simulink model "model_for_IM_with_ITSC_fault"  (R2016a)
settings: Solver=VariableStepAuto  StartTime=0.0  StopTime=2  FixedStep=2e-6  MaxStep=2e-6  RelTol=1e-6
libraries: powerlib x34, powerlib_meascontrol x1
settings Model: Creator=Pietro  LastModifiedBy=silker
settings SolverCC: ZeroCrossControl=DisableAll
settings DataIOCC: LimitDataPoints=on  SaveFormat=Array  SignalLoggingSaveFormat=ModelDataLogs
settings OptimizationCC: ExpressionDepthLimit=2147483647  InitFltsAndDblsToZero=on
settings DebuggingCC: SaveWithParameterizedLinksMsg=none  UnderspecifiedInitializationDetection=Classic  MergeDetectMultiDrivingBlocksExec=none  SignalResolutionControl=TryResolveAllWithWarning  SolverPrmCheckMsg=warning  MultiTaskDSMMsg=warning  MultiTaskCondExecSysMsg=none  FcnCallInpInsideContextMsg=UseLocalSettings  StateNameClashWarn=warning
settings HardwareCC: ProdBitPerPointer=32  ProdLargestAtomicFloat=None  ProdIntDivRoundTo=Undefined  ProdEndianess=Unspecified  ProdWordSize=32  ProdHWDeviceType=32-bit Generic
settings ModelReferenceCC: PropagateSignalLabelsOutOfModel=off
settings GRTTargetCC: TargetFcnLib=ansi_tfl_tmw.mat  CombineOutputUpdateFcns=off  GRTInterface=on
settings ConfigComp: CovModelRefEnable=Off

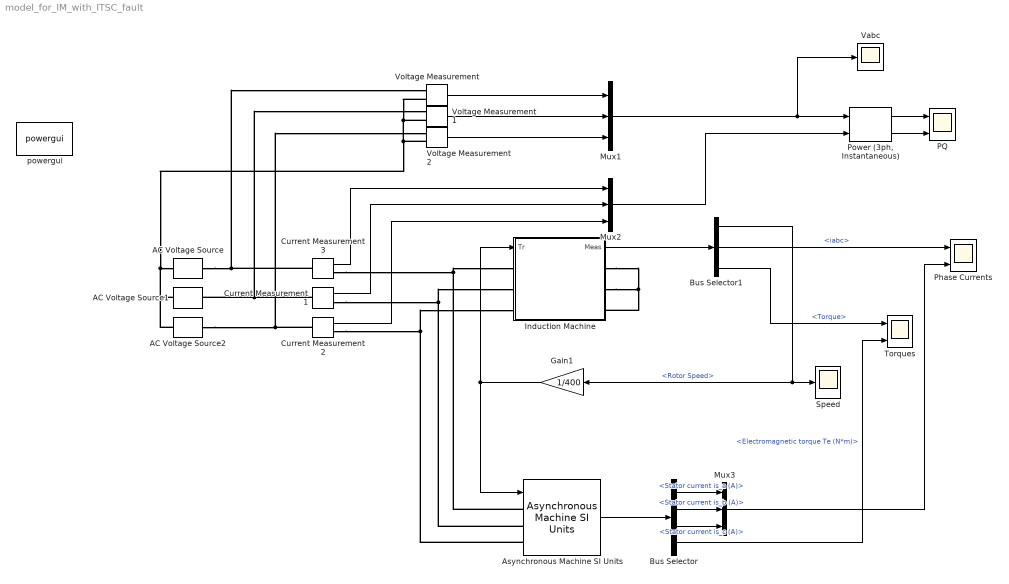
== system model_for_IM_with_ITSC_fault ==
  AC Voltage Source : powerlib/Electrical Sources/AC Voltage Source  Amplitude=80  Phase=0  Frequency=50  SampleTime=-1  Measurements=None  BusType=swing  Pref=10e3  Qref=0  Qmin=-inf  Qmax=+inf
  AC Voltage Source1 : powerlib/Electrical Sources/AC Voltage Source  Amplitude=80  Phase=240  Frequency=50  SampleTime=-1  Measurements=None  BusType=swing  Pref=10e3  Qref=0  Qmin=-inf  Qmax=+inf
  AC Voltage Source2 : powerlib/Electrical Sources/AC Voltage Source  Amplitude=80  Phase=120  Frequency=50  SampleTime=-1  Measurements=None  BusType=swing  Pref=10e3  Qref=0  Qmin=-inf  Qmax=+inf
  Asynchronous Machine SI Units : powerlib/Machines/Asynchronous Machine SI Units  RotorType=Squirrel-cage  PresetModel=No  MechanicalLoad=Torque Tm  ShowDetailedParameters=on  ReferenceFrame=Rotor  Units=SI  MeasurementBus=off  NominalParameters=[500 150 50]  Stator=[2.3 0.005]  Rotor=[3.1 0.001]  Cage1=[0.4155 0.002066]  Cage2=[0.4168 0.0003495]  Lm=0.090  Mechanical=[0.005 0.0000001 1]  PolePairs=2  InitialConditions=[1 0 0 0 0 0 0 0]  SimulateSaturation=off  Saturation=[14.03593122, 27.81365428, 53.79336849, 72.68890987, 97.98006896, 148.6815601, 215.7428561, 302.9841135, 428.7778367 ; 230, 322, 414, 460, 506, 552, 598, 644, 690]  LoadFlowParameters=1492000  TsPowergui=0  TsBlock=-1  IterativeModel=Trapezoidal non iterative  IterativeDiscreteModel=Trapezoidal non iterative  Pmec=1.492e+006
  Bus Selector : BusSelector  OutputSignals=Stator measurements.Stator current is_a (A),Stator measurements.Stator current is_b (A),Stator measurements.Stator current is_c (A),Mechanical.Electromagnetic torque Te (N*m)
  Bus Selector1 : BusSelector  OutputSignals=Rotor Speed,iabc,Torque
  Current Measurement1 : powerlib/Measurements/Current Measurement  PhasorSimulation=off  OutputType=Complex  PSBequivalent=0
  Current Measurement2 : powerlib/Measurements/Current Measurement  PhasorSimulation=off  OutputType=Complex  PSBequivalent=0
  Current Measurement3 : powerlib/Measurements/Current Measurement  PhasorSimulation=off  OutputType=Complex  PSBequivalent=0
  Gain1 : Gain  Gain=1/400
  Induction Machine : Subsystem  mask{Rs=2.3, Rr=3.1, Lm=0.090, Lls=0.005, Llr=0.001, PP=1, J=0.005, Kf=0.05, Rf=0.20}
      mask prompts: Kf "Fault Ratio"; Rf "Fault Resistance"
      mask help:
      | The initial VBR-based IM model by Pietro Tricoli,
      | Original file downloaded from:
      | https://www.mathworks.com/matlabcentral/fileexchange/53174-induction-machine-model
      mask init:
      | Lr=Llr+Lm;
      | Ls=Lls+Lm;
  Mux1 : Mux  Inputs=3
  Mux2 : Mux  Inputs=3
  Mux3 : Mux  Inputs=3
  PQ : Scope  NumInputPorts=2
  Phase Currents : Scope  NumInputPorts=2
  "Power (3ph, Instantaneous)" : powerlib_meascontrol/Measurements/Power (3ph, Instantaneous)
  Speed : Scope
  Torques : Scope  NumInputPorts=2
  Vabc : Scope
  Voltage Measurement : powerlib/Measurements/Voltage Measurement  PhasorSimulation=off  OutputType=Complex  PSBequivalent=0
  Voltage Measurement1 : powerlib/Measurements/Voltage Measurement  PhasorSimulation=off  OutputType=Complex  PSBequivalent=0
  Voltage Measurement2 : powerlib/Measurements/Voltage Measurement  PhasorSimulation=off  OutputType=Complex  PSBequivalent=0
  powergui : powerlib/powergui  Priority=1  SimulationMode=Discrete  SolverType=Tustin  SampleTime=2e-6  frequency=60  SPID=off  DisableSnubberDevices=off  DisableRonSwitches=off  DisableVfSwitches=off  SwTol=0  DisplayEquations=off  Interpol=off  ExternalGateDelay=off  methode=off  Ts=10  FunctionMessages=off  echomessages=off  HookPort=off  EnableUseOfTLC=off  x0status=blocks  frequencyindice=0  Pbase=100e6  ErrMax=1e-4  Iterations=50  UnitsV=kV  UnitsW=MW  buscounter=0  RestoreLinks=warning  ResistiveCurrentMeasurement=off  Frange=[0:2:500]  Ylog=off  Xlog=on  ShowGrid=off  save=off  variable=ZData  structure=0  ZoomFFT=off  StartTime=0.0  cycles=1  DisplayStyle=1  fundamental=60  FreqAxis=off  MaxFrequency=1000  frequencyindicesteady=1  RmsSteady=1  display=off
  wires:
  Voltage Measurement/1 -> Mux1/1
  Asynchronous Machine SI Units/1 -> Bus Selector/1
  Induction Machine/1(Meas) -> Bus Selector1/1
  Bus Selector1/1 -> Gain1/1, Speed/1  "<Rotor Speed>"
  Bus Selector1/2 -> Phase Currents/1  "<iabc>"
  Gain1/1 -> Asynchronous Machine SI Units/1, Induction Machine/1(Tr)
  Voltage Measurement1/1 -> Mux1/2
  Voltage Measurement2/1 -> Mux1/3
  Current Measurement3/1 -> Mux2/1
  Current Measurement1/1 -> Mux2/2
  Current Measurement2/1 -> Mux2/3
  Mux1/1 -> Vabc/1, "Power (3ph, Instantaneous)"/1
  Mux2/1 -> "Power (3ph, Instantaneous)"/2
  "Power (3ph, Instantaneous)"/1 -> PQ/1
  "Power (3ph, Instantaneous)"/2 -> PQ/2
  Bus Selector1/3 -> Torques/1  "<Torque>"
  Bus Selector/4 -> Torques/2  "<Electromagnetic torque Te (N*m)>"
  Bus Selector/2 -> Mux3/2  "<Stator current is_b (A)>"
  Bus Selector/1 -> Mux3/1  "<Stator current is_a (A)>"
  Bus Selector/3 -> Mux3/3  "<Stator current is_c (A)>"
  Mux3/1 -> Phase Currents/2
  connections:
  Asynchronous Machine SI Units/LConn2 -- Current Measurement1/RConn1 -- Induction Machine/LConn2
  Asynchronous Machine SI Units/LConn3 -- Current Measurement2/RConn1 -- Induction Machine/LConn3
  Asynchronous Machine SI Units/LConn1 -- Current Measurement3/RConn1 -- Induction Machine/LConn1
  Induction Machine/RConn1 -- Induction Machine/RConn3 -- Induction Machine/RConn2
  AC Voltage Source2/RConn1 -- Current Measurement2/LConn1 -- Voltage Measurement2/LConn1
  Current Measurement1/LConn1 -- AC Voltage Source1/RConn1 -- Voltage Measurement1/LConn1
  AC Voltage Source/RConn1 -- Current Measurement3/LConn1 -- Voltage Measurement/LConn1
  AC Voltage Source2/LConn1 -- AC Voltage Source1/LConn1 -- Voltage Measurement/LConn2 -- Voltage Measurement1/LConn2 -- Voltage Measurement2/LConn2 -- AC Voltage Source/LConn1

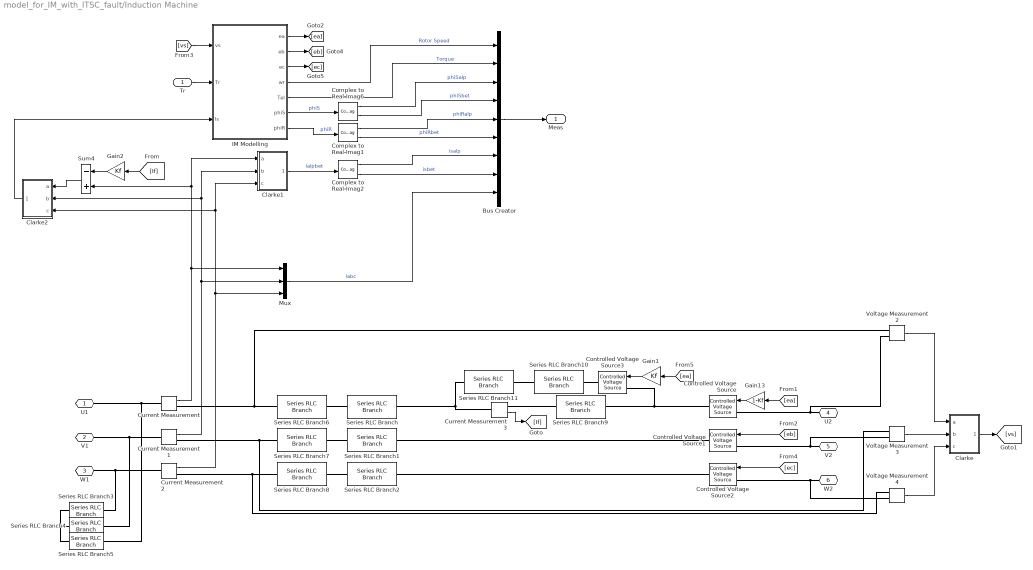
== system model_for_IM_with_ITSC_fault/Induction Machine ==
  Tr : Inport
  Bus Creator : BusCreator  Inputs=9
  Clarke : Subsystem
  Clarke1 : Subsystem
  Clarke2 : Subsystem
  Complex to Real-Imag1 : ComplexToRealImag
  Complex to Real-Imag2 : ComplexToRealImag
  Complex to Real-Imag6 : ComplexToRealImag
  Controlled Voltage Source{,1..3} (4 alike) : powerlib/Electrical Sources/Controlled Voltage Source  Initialize=on  Source_Type=AC  Amplitude=0  Phase=0  Frequency=0  Measurements=None
  Current Measurement{,1..3} (4 alike) : powerlib/Measurements/Current Measurement  PhasorSimulation=off  OutputType=Complex  PSBequivalent=0
  Gain1 : Gain  Gain=Kf
  Gain13 : Gain  Gain=1-Kf
  Gain2 : Gain  Gain=Kf
  IM Modelling : Subsystem
  Mux : Mux  Inputs=3
  Series RLC Branch : powerlib/Elements/Series RLC Branch  LConnTagsString=__new0  RConnTagsString=__new0  BranchType=L  Resistance=Rs  Inductance=Lls*(1-Kf)  SetiL0=off  InitialCurrent=0  Capacitance=1e-6  Setx0=off  InitialVoltage=0  Measurements=None
  Series RLC Branch1 : powerlib/Elements/Series RLC Branch  LConnTagsString=__new0  RConnTagsString=__new0  BranchType=L  Resistance=Rs  Inductance=Lls  SetiL0=on  InitialCurrent=0  Capacitance=1e-6  Setx0=off  InitialVoltage=0  Measurements=None
  Series RLC Branch10 : powerlib/Elements/Series RLC Branch  LConnTagsString=__new0  RConnTagsString=__new0  BranchType=L  Resistance=Rs  Inductance=Lls*Kf  SetiL0=off  InitialCurrent=0  Capacitance=1e-6  Setx0=off  InitialVoltage=0  Measurements=None
  Series RLC Branch11 : powerlib/Elements/Series RLC Branch  LConnTagsString=__new0  RConnTagsString=__new0  BranchType=R  Resistance=Rs*Kf  Inductance=Lls  SetiL0=off  InitialCurrent=0  Capacitance=1e-6  Setx0=off  InitialVoltage=0  Measurements=None
  Series RLC Branch2 : powerlib/Elements/Series RLC Branch  LConnTagsString=__new0  RConnTagsString=__new0  BranchType=L  Resistance=Rs  Inductance=Lls  SetiL0=on  InitialCurrent=0  Capacitance=1e-6  Setx0=off  InitialVoltage=0  Measurements=None
  Series RLC Branch3 : powerlib/Elements/Series RLC Branch  LConnTagsString=__new0  RConnTagsString=__new0  BranchType=R  Resistance=1e12  Inductance=Lls  SetiL0=off  InitialCurrent=0  Capacitance=1e-6  Setx0=off  InitialVoltage=0  Measurements=None
  Series RLC Branch4 : powerlib/Elements/Series RLC Branch  LConnTagsString=__new0  RConnTagsString=__new0  BranchType=R  Resistance=1e12  Inductance=Lls  SetiL0=off  InitialCurrent=0  Capacitance=1e-6  Setx0=off  InitialVoltage=0  Measurements=None
  Series RLC Branch5 : powerlib/Elements/Series RLC Branch  LConnTagsString=__new0  RConnTagsString=__new0  BranchType=R  Resistance=1e12  Inductance=Lls  SetiL0=off  InitialCurrent=0  Capacitance=1e-6  Setx0=off  InitialVoltage=0  Measurements=None
  Series RLC Branch6 : powerlib/Elements/Series RLC Branch  LConnTagsString=__new0  RConnTagsString=__new0  BranchType=R  Resistance=Rs*(1-Kf)  Inductance=Lls  SetiL0=off  InitialCurrent=0  Capacitance=1e-6  Setx0=off  InitialVoltage=0  Measurements=None
  Series RLC Branch7 : powerlib/Elements/Series RLC Branch  LConnTagsString=__new0  RConnTagsString=__new0  BranchType=R  Resistance=Rs  Inductance=Lls  SetiL0=on  InitialCurrent=0  Capacitance=1e-6  Setx0=off  InitialVoltage=0  Measurements=None
  Series RLC Branch8 : powerlib/Elements/Series RLC Branch  LConnTagsString=__new0  RConnTagsString=__new0  BranchType=R  Resistance=Rs  Inductance=Lls  SetiL0=on  InitialCurrent=0  Capacitance=1e-6  Setx0=off  InitialVoltage=0  Measurements=None
  Series RLC Branch9 : powerlib/Elements/Series RLC Branch  LConnTagsString=__new0  RConnTagsString=__new0  BranchType=R  Resistance=Rf  Inductance=Lls  SetiL0=on  InitialCurrent=0  Capacitance=1e-6  Setx0=off  InitialVoltage=0  Measurements=None
  Sum4 : Sum  Inputs=-+
  Voltage Measurement2 : powerlib/Measurements/Voltage Measurement  PhasorSimulation=off  OutputType=Complex  PSBequivalent=0
  Voltage Measurement3 : powerlib/Measurements/Voltage Measurement  PhasorSimulation=off  OutputType=Complex  PSBequivalent=0
  Voltage Measurement4 : powerlib/Measurements/Voltage Measurement  PhasorSimulation=off  OutputType=Complex  PSBequivalent=0
  U1 : PMIOPort  Port=1  Side=Left
  V1 : PMIOPort  Port=2  Side=Left
  W1 : PMIOPort  Port=3  Side=Left
  U2 : PMIOPort  Port=4  Side=Right
  V2 : PMIOPort  Port=5  Side=Right
  W2 : PMIOPort  Port=6  Side=Right
  Meas : Outport
  wires:
  Tr/1 -> IM Modelling/2(Tr)
  [eb] -> Controlled Voltage Source1/1
  Current Measurement1/1 -> Clarke2/2(b), Clarke1/2(b), Mux/2
  Current Measurement/1 -> Clarke1/1(a), Sum4/2, Mux/1
  IM Modelling/1(ea) -> [ea]
  IM Modelling/2(eb) -> [eb]
  IM Modelling/3(ec) -> [ec]
  IM Modelling/4(wr) -> Bus Creator/1  "Rotor Speed"
  [vs] -> IM Modelling/1(vs)
  Voltage Measurement2/1 -> Clarke/1(a)
  Voltage Measurement3/1 -> Clarke/2(b)
  Voltage Measurement4/1 -> Clarke/3(c)
  Clarke/1(alp bet) -> [vs]
  IM Modelling/5(Tel) -> Bus Creator/2  "Torque"
  Bus Creator/1 -> Meas/1
  Complex to Real-Imag6/1 -> Bus Creator/3  "phiSalp"
  Complex to Real-Imag6/2 -> Bus Creator/4  "phiSbet"
  IM Modelling/6(phiS) -> Complex to Real-Imag6/1  "phiS"
  IM Modelling/7(phiR) -> Complex to Real-Imag1/1  "phiR"
  Complex to Real-Imag1/1 -> Bus Creator/5  "phiRalp"
  Complex to Real-Imag1/2 -> Bus Creator/6  "phiRbet"
  Clarke1/1(alp bet) -> Complex to Real-Imag2/1  "ialpbet"
  Complex to Real-Imag2/1 -> Bus Creator/7  "isalp"
  Complex to Real-Imag2/2 -> Bus Creator/8  "isbet"
  Mux/1 -> Bus Creator/9  "iabc"
  Gain1/1 -> Controlled Voltage Source3/1
  Gain13/1 -> Controlled Voltage Source/1
  [ea] -> Gain13/1
  [ec] -> Controlled Voltage Source2/1
  Current Measurement3/1 -> [If]
  [ea] -> Gain1/1
  Current Measurement2/1 -> Clarke1/3(c), Clarke2/3(c), Mux/3
  Sum4/1 -> Clarke2/1(a)
  Gain2/1 -> Sum4/1
  [If] -> Gain2/1
  Clarke2/1(alp bet) -> IM Modelling/3(Is)
  connections:
  Controlled Voltage Source1/RConn1 -- Series RLC Branch1/RConn1
  U1/RConn1 -- Series RLC Branch5/RConn1 -- Current Measurement/LConn1
  Current Measurement1/LConn1 -- Series RLC Branch4/RConn1 -- V1/RConn1
  Current Measurement2/LConn1 -- Series RLC Branch3/RConn1 -- W1/RConn1
  V2/RConn1 -- Voltage Measurement3/LConn2 -- Controlled Voltage Source1/LConn1
  W2/RConn1 -- Voltage Measurement4/LConn2 -- Controlled Voltage Source2/LConn1
  Controlled Voltage Source/LConn1 -- Voltage Measurement2/LConn2 -- U2/RConn1
  Series RLC Branch3/LConn1 -- Series RLC Branch4/LConn1 -- Series RLC Branch5/LConn1
  Series RLC Branch8/RConn1 -- Series RLC Branch2/LConn1
  Series RLC Branch7/RConn1 -- Series RLC Branch1/LConn1
  Series RLC Branch6/RConn1 -- Series RLC Branch/LConn1
  Series RLC Branch6/LConn1 -- Current Measurement/RConn1 -- Voltage Measurement2/LConn1
  Series RLC Branch7/LConn1 -- Voltage Measurement3/LConn1 -- Current Measurement1/RConn1
  Series RLC Branch8/LConn1 -- Current Measurement2/RConn1 -- Voltage Measurement4/LConn1
  Series RLC Branch9/RConn1 -- Controlled Voltage Source/RConn1 -- Controlled Voltage Source3/LConn1
  Controlled Voltage Source2/RConn1 -- Series RLC Branch2/RConn1
  Series RLC Branch11/RConn1 -- Series RLC Branch10/LConn1
  Controlled Voltage Source3/RConn1 -- Series RLC Branch10/RConn1
  Current Measurement3/LConn1 -- Series RLC Branch/RConn1 -- Series RLC Branch11/LConn1
  Current Measurement3/RConn1 -- Series RLC Branch9/LConn1

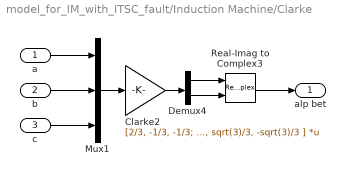
== system model_for_IM_with_ITSC_fault/Induction Machine/Clarke ==
  a : Inport
  b : Inport  Port=2
  c : Inport  Port=3
  Clarke2 : Gain  Gain=[2/3, -1/3, -1/3; 0, sqrt(3)/3, -sqrt(3)/3 ]  Multiplication=Matrix(K*u)
  Demux4 : Demux  Outputs=2
  Mux1 : Mux  Inputs=3
  Real-Imag to Complex3 : RealImagToComplex
  alp bet : Outport
  wires:
  Mux1/1 -> Clarke2/1
  Clarke2/1 -> Demux4/1
  a/1 -> Mux1/1
  Demux4/1 -> Real-Imag to Complex3/1
  Real-Imag to Complex3/1 -> alp bet/1
  Demux4/2 -> Real-Imag to Complex3/2
  c/1 -> Mux1/3
  b/1 -> Mux1/2

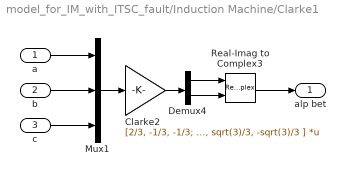
== system model_for_IM_with_ITSC_fault/Induction Machine/Clarke1 ==
  a : Inport
  b : Inport  Port=2
  c : Inport  Port=3
  Clarke2 : Gain  Gain=[2/3, -1/3, -1/3; 0, sqrt(3)/3, -sqrt(3)/3 ]  Multiplication=Matrix(K*u)
  Demux4 : Demux  Outputs=2
  Mux1 : Mux  Inputs=3
  Real-Imag to Complex3 : RealImagToComplex
  alp bet : Outport
  wires:
  Mux1/1 -> Clarke2/1
  Clarke2/1 -> Demux4/1
  a/1 -> Mux1/1
  Demux4/1 -> Real-Imag to Complex3/1
  Real-Imag to Complex3/1 -> alp bet/1
  Demux4/2 -> Real-Imag to Complex3/2
  c/1 -> Mux1/3
  b/1 -> Mux1/2

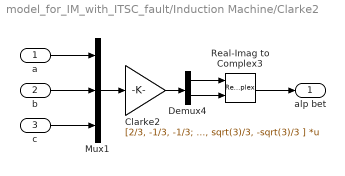
== system model_for_IM_with_ITSC_fault/Induction Machine/Clarke2 ==
  a : Inport
  b : Inport  Port=2
  c : Inport  Port=3
  Clarke2 : Gain  Gain=[2/3, -1/3, -1/3; 0, sqrt(3)/3, -sqrt(3)/3 ]  Multiplication=Matrix(K*u)
  Demux4 : Demux  Outputs=2
  Mux1 : Mux  Inputs=3
  Real-Imag to Complex3 : RealImagToComplex
  alp bet : Outport
  wires:
  b/1 -> Mux1/2
  c/1 -> Mux1/3
  Demux4/2 -> Real-Imag to Complex3/2
  Real-Imag to Complex3/1 -> alp bet/1
  Demux4/1 -> Real-Imag to Complex3/1
  a/1 -> Mux1/1
  Clarke2/1 -> Demux4/1
  Mux1/1 -> Clarke2/1

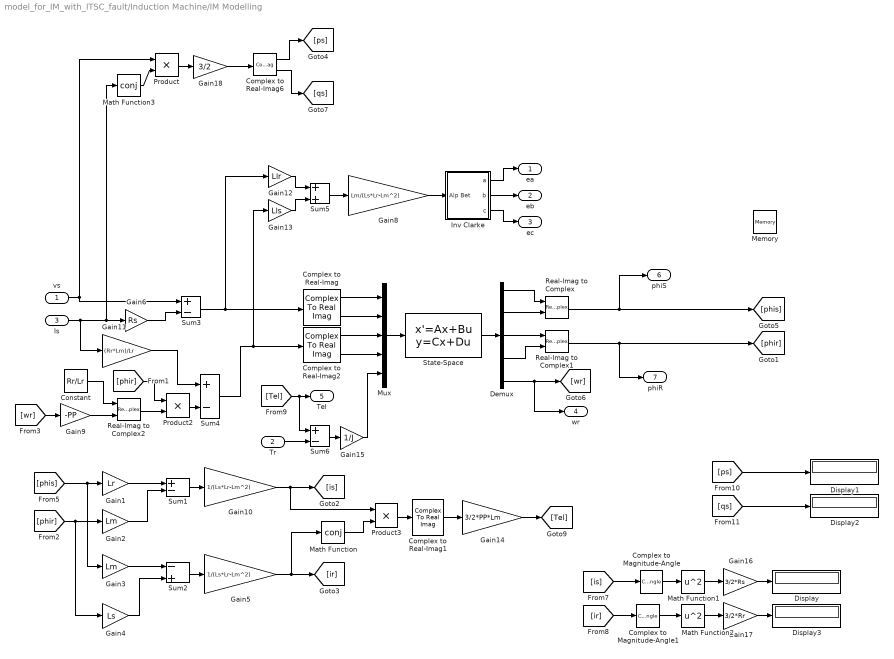
== system model_for_IM_with_ITSC_fault/Induction Machine/IM Modelling ==
  vs : Inport
  Tr : Inport  Port=2
  Is : Inport  Port=3
  Complex to Magnitude-Angle : ComplexToMagnitudeAngle  Output=Magnitude
  Complex to Magnitude-Angle1 : ComplexToMagnitudeAngle  Output=Magnitude
  Complex to Real-Imag : ComplexToRealImag
  Complex to Real-Imag1 : ComplexToRealImag  Output=Imag
  Complex to Real-Imag2 : ComplexToRealImag
  Complex to Real-Imag6 : ComplexToRealImag
  Constant : Constant  Value=Rr/Lr
  Demux : Demux  Outputs=5
  Display{,1..3} (4 alike) : Display
  Gain1 : Gain  Gain=Lr
  Gain10 : Gain  Gain=1/(Ls*Lr-Lm^2)
  Gain11 : Gain  Gain=(Rr*Lm)/Lr
  Gain12 : Gain  Gain=Llr
  Gain13 : Gain  Gain=Lls
  Gain14 : Gain  Gain=3/2*PP*Lm
  Gain15 : Gain  Gain=1/J
  Gain16 : Gain  Gain=3/2*Rs
  Gain17 : Gain  Gain=3/2*Rr
  Gain18 : Gain  Gain=3/2
  Gain2 : Gain  Gain=Lm
  Gain3 : Gain  Gain=Lm
  Gain4 : Gain  Gain=Ls
  Gain5 : Gain  Gain=1/(Ls*Lr-Lm^2)
  Gain6 : Gain  Gain=Rs
  Gain8 : Gain  Gain=Lm/(Ls*Lr-Lm^2)
  Gain9 : Gain  Gain=-PP
  Inv Clarke : Subsystem
  Math Function : Math  Operator=conj  SaturateOnIntegerOverflow=on
  Math Function1 : Math  Operator=square  SaturateOnIntegerOverflow=on
  Math Function2 : Math  Operator=square  SaturateOnIntegerOverflow=on
  Math Function3 : Math  Operator=conj  SaturateOnIntegerOverflow=on
  Memory : Memory  InheritSampleTime=on
  Mux : Mux  Inputs=5
  Product : Product  RndMeth=Zero
  Product2 : Product  RndMeth=Zero
  Product3 : Product  RndMeth=Zero
  Real-Imag to Complex : RealImagToComplex
  Real-Imag to Complex1 : RealImagToComplex
  Real-Imag to Complex2 : RealImagToComplex
  State-Space : StateSpace  A=[0,0,0,0,0; 0,0,0,0,0; 0,0,0,0,0; 0,0,0,0,0; 0,0,0,0,0]  B=[1,0,0,0,0; 0,1,0,0,0; 0,0,1,0,0; 0,0,0,1,0; 0,0,0,0,1]  C=[1,0,0,0,0; 0,1,0,0,0; 0,0,1,0,0; 0,0,0,1,0; 0,0,0,0,1]  D=[0,0,0,0,0; 0,0,0,0,0; 0,0,0,0,0; 0,0,0,0,0; 0,0,0,0,0]  X0=[0,0,0,0,0]
  Sum{1,3..4,6} (4 alike) : Sum  Inputs=+-
  Sum2 : Sum  Inputs=-+
  Sum5 : Sum
  ea : Outport
  eb : Outport  Port=2
  ec : Outport  Port=3
  wr : Outport  Port=4
  Tel : Outport  Port=5
  phiS : Outport  Port=6
  phiR : Outport  Port=7
  wires:
  Demux/1 -> Real-Imag to Complex/1
  Demux/2 -> Real-Imag to Complex/2
  Complex to Real-Imag/1 -> Mux/1
  Complex to Real-Imag/2 -> Mux/2
  Gain14/1 -> [Tel]
  Sum6/1 -> Gain15/1
  [Tel] -> Sum6/1, Tel/1
  Tr/1 -> Sum6/2
  Demux/5 -> wr/1, [wr]
  Demux/3 -> Real-Imag to Complex1/1
  Demux/4 -> Real-Imag to Complex1/2
  Gain15/1 -> Mux/5
  [phis] -> Gain1/1, Gain3/1
  Gain1/1 -> Sum1/1
  Gain2/1 -> Sum1/2
  [phir] -> Gain4/1, Gain2/1
  Sum1/1 -> Gain10/1
  Gain3/1 -> Sum2/1
  Gain4/1 -> Sum2/2
  Sum2/1 -> Gain5/1
  Complex to Real-Imag2/1 -> Mux/3
  Complex to Real-Imag2/2 -> Mux/4
  Gain5/1 -> Math Function/1, [ir]
  Complex to Real-Imag1/1 -> Gain14/1
  Product3/1 -> Complex to Real-Imag1/1
  Math Function/1 -> Product3/2
  Is/1 -> Gain11/1, Math Function3/1, Gain6/1
  vs/1 -> Product/1, Sum3/1
  Sum5/1 -> Gain8/1
  Gain13/1 -> Sum5/2
  Gain12/1 -> Sum5/1
  [is] -> Complex to Magnitude-Angle/1
  Complex to Magnitude-Angle/1 -> Math Function1/1
  Math Function1/1 -> Gain16/1
  Gain16/1 -> Display/1
  [ir] -> Complex to Magnitude-Angle1/1
  Complex to Magnitude-Angle1/1 -> Math Function2/1
  Math Function2/1 -> Gain17/1
  Gain17/1 -> Display3/1
  [ps] -> Display1/1
  [qs] -> Display2/1
  Product/1 -> Gain18/1
  Math Function3/1 -> Product/2
  Gain18/1 -> Complex to Real-Imag6/1
  Complex to Real-Imag6/1 -> [ps]
  Complex to Real-Imag6/2 -> [qs]
  Mux/1 -> State-Space/1
  Gain8/1 -> Inv Clarke/1(Alp Bet)
  Inv Clarke/3(c) -> ec/1
  Inv Clarke/1(a) -> ea/1
  Inv Clarke/2(b) -> eb/1
  State-Space/1 -> Demux/1
  Gain10/1 -> Product3/1, [is]
  [wr] -> Gain9/1
  Gain9/1 -> Real-Imag to Complex2/2
  Constant/1 -> Real-Imag to Complex2/1
  Real-Imag to Complex2/1 -> Product2/2
  [phir] -> Product2/1
  Product2/1 -> Sum4/2
  Gain11/1 -> Sum4/1
  Sum4/1 -> Gain13/1, Complex to Real-Imag2/1
  Real-Imag to Complex/1 -> [phis], phiS/1
  Real-Imag to Complex1/1 -> [phir], phiR/1
  Gain6/1 -> Sum3/2
  Sum3/1 -> Gain12/1, Complex to Real-Imag/1

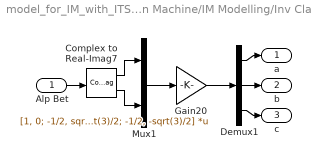
== system model_for_IM_with_ITSC_fault/Induction Machine/IM Modelling/Inv Clarke ==
  Alp Bet : Inport
  Complex to Real-Imag7 : ComplexToRealImag
  Demux1 : Demux  Outputs=3
  Gain20 : Gain  Gain=[1, 0; -1/2, sqrt(3)/2; -1/2, -sqrt(3)/2]  Multiplication=Matrix(K*u)
  Mux1 : Mux  Inputs=2
  a : Outport
  b : Outport  Port=2
  c : Outport  Port=3
  wires:
  Mux1/1 -> Gain20/1
  Complex to Real-Imag7/2 -> Mux1/2
  Alp Bet/1 -> Complex to Real-Imag7/1
  Demux1/2 -> b/1
  Demux1/3 -> c/1
  Gain20/1 -> Demux1/1
  Demux1/1 -> a/1
  Complex to Real-Imag7/1 -> Mux1/1
